simulink model "acc"  (R2020a)
settings: Solver=VariableStepAuto  StartTime=0.0  StopTime=inf  RelTol=1e-3
settings Model: Creator=shesh  LastModifiedBy=shesh

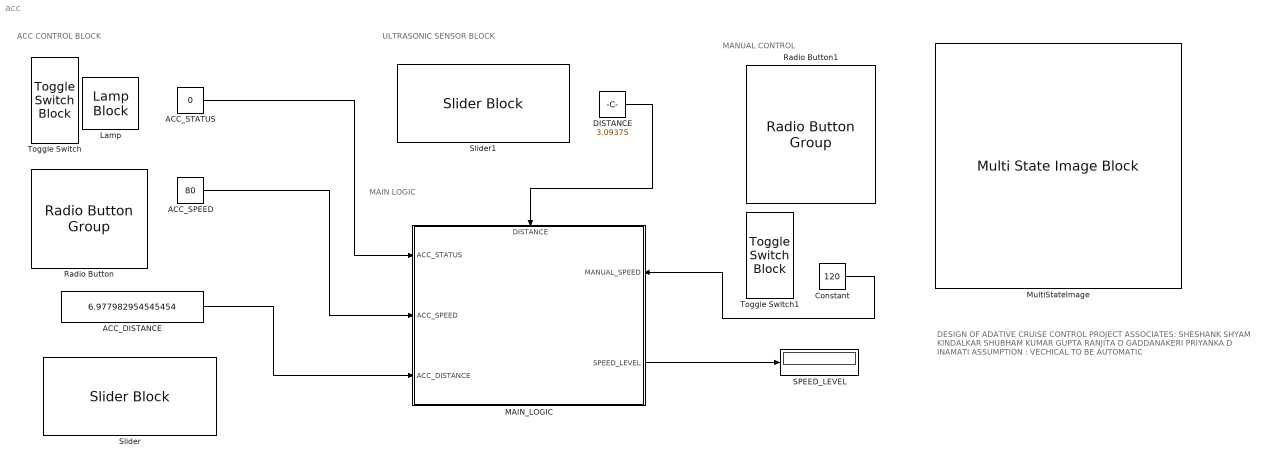
== system acc ==
  note: DESIGN OF ADATIVE CRUISE CONTROL
      |
      | PROJECT ASSOCIATES:
      | SHESHANK SHYAM KINDALKAR
      | SHUBHAM KUMAR GUPTA
      | RANJITA D GADDANAKERI
      | PRIYANKA D INAMATI
      |
      | ASSUMPTION : VECHICAL TO BE AUTOMATIC
  note: MANUAL CONTROL
  note: MAIN LOGIC
  note: ULTRASONIC SENSOR BLOCK
  note: ACC CONTROL BLOCK
  ACC_DISTANCE : Constant  Value=6.977982954545454  OutMin=[0]  OutMax=[10]
  ACC_SPEED : Constant  Value=80
  ACC_STATUS : Constant  Value=0
  Constant : Constant  Value=120
  DISTANCE : Constant  Value=3.09375
  Lamp : LampBlock
  MAIN_LOGIC : Stateflow chart  TreatAsAtomicUnit=on
      settings: PortSchema="{\"entries\":[{\"content\":{\"sides\":[{\"content\":{\"connectorIds\":[\"In3\",\"In4\",\"In5\"]},\"type\":\"ConnectorPlacement.EquallySpacedRectSide\",\"uuid\":\"9577933f-3cd5-4877-b3f1-1cabc5f66bc2\"},{\"content\":{\"connectorIds\":[\"In1\",\"Out1\"],\"side\":\"RIGHT\"},\"type\":\"ConnectorPlacement.EquallySpacedRectSide\",\"uuid\":\"2a6dc85d-fd72-47ef-ac66-14217eaecbf8\"},{\"content\":{\"connectorIds\":[\"In2\"],\"side\":\"TOP\"},\"type\":\"ConnectorPlacement.EquallySpacedRectSide\",\"uuid\":\"38d285f4-ccf6-4804-ae1f-6877806054a5\"}]},\"type\":\"ConnectorPlacement.EquallySpacedConnector\",\"uuid\":\"df4108ed-a8cc-4829-9830-7e09486e0f89\"}],\"packageUris\":[\"http://schema.mathworks.com/mf0/Connector/19700101\"],\"version\":\"1.0\"}"
  MultiStateImage : MultiStateImageBlock
  Radio Button : RadioButtonGroup  SelectedLabel=80 KMPH  ButtonGroupName=Group
      settings: Values={{'30 KMPH', '50 KMPH', '80 KMPH', '100 KMPH'}, [30 50 80 100]}
  Radio Button1 : RadioButtonGroup  SelectedLabel=120 KMPH  ButtonGroupName=Group
      settings: Values={{'40 KMPH', '80 KMPH', '120 KMPH', '160 KMPH', 'BREAK'}, [40 80 120 160 0]}
  SPEED_LEVEL : Display
  Slider : SliderBlock  ScaleMin=5  ScaleMax=10  TickInterval=1
  Slider1 : SliderBlock  ScaleMax=20
  Toggle Switch : ToggleSwitchBlock
      settings: Values={{'Off', 'On'}, [0 1]}
  Toggle Switch1 : ToggleSwitchBlock
      settings: Values={{'Off', 'On'}, [1 0]}
  wires:
  ACC_STATUS/1 -> MAIN_LOGIC/3(ACC_STATUS)
  ACC_SPEED/1 -> MAIN_LOGIC/4(ACC_SPEED)
  ACC_DISTANCE/1 -> MAIN_LOGIC/5(ACC_DISTANCE)
  DISTANCE/1 -> MAIN_LOGIC/2(DISTANCE)
  MAIN_LOGIC/1(SPEED_LEVEL) -> SPEED_LEVEL/1
  Constant/1 -> MAIN_LOGIC/1(MANUAL_SPEED)

== stateflow chart acc/MAIN_LOGIC ==
  state ADAPTIVE_CONTROL_ACTIVE
    entry:
    state ZERO_GEAR_STATE
      entry:
      SPEED_LEVEL = 0;
    state FRIST_GEAR_STATE
      entry:
      SPEED_LEVEL = 1;
    state SECOND_GEAR_STATE
      entry:
      SPEED_LEVEL = 2;
    state BREAKING_STATE
      entry:
      SPEED_LEVEL = 3;
    (default) -> ZERO_GEAR_STATE
    SECOND_GEAR_STATE -> FRIST_GEAR_STATE [order 5] : [ACC_SPEED == 80]
    ZERO_GEAR_STATE -> FRIST_GEAR_STATE [order 2] : [DISTANCE >= 0.20*ACC_DISTANCE]
    ZERO_GEAR_STATE -> ADAPTIVE_CONTROL_ACTIVE.BREAKING_STATE [order 1] : [DISTANCE >= 0.75*ACC_DISTANCE]
    FRIST_GEAR_STATE -> ZERO_GEAR_STATE [order 3] : [ACC_SPEED == 30 || ACC_SPEED == 50]
    ZERO_GEAR_STATE -> FRIST_GEAR_STATE [order 3] : [ACC_SPEED == 80]
    ADAPTIVE_CONTROL_ACTIVE.BREAKING_STATE -> FRIST_GEAR_STATE [order 4] : [ACC_SPEED == 80]
    FRIST_GEAR_STATE -> SECOND_GEAR_STATE [order 4] : [ACC_SPEED == 100]
    SECOND_GEAR_STATE -> ZERO_GEAR_STATE [order 4] : [ACC_SPEED == 30 || ACC_SPEED == 50]
    SECOND_GEAR_STATE -> ZERO_GEAR_STATE [order 2] : [DISTANCE >= 0.50*ACC_DISTANCE]
    ZERO_GEAR_STATE -> SECOND_GEAR_STATE [order 4] : [ACC_SPEED == 100]
    ADAPTIVE_CONTROL_ACTIVE.BREAKING_STATE -> ZERO_GEAR_STATE [order 1] : [DISTANCE >= 0.50*ACC_DISTANCE]
    ADAPTIVE_CONTROL_ACTIVE.BREAKING_STATE -> ZERO_GEAR_STATE [order 3] : [ACC_SPEED == 30 || ACC_SPEED == 50]
    FRIST_GEAR_STATE -> ZERO_GEAR_STATE [order 2] : [DISTANCE >= 0.50*ACC_DISTANCE]
    SECOND_GEAR_STATE -> FRIST_GEAR_STATE [order 3] : [DISTANCE >= 0.20*ACC_DISTANCE]
    FRIST_GEAR_STATE -> ADAPTIVE_CONTROL_ACTIVE.BREAKING_STATE [order 1] : [DISTANCE >= 0.75*ACC_DISTANCE]
    ADAPTIVE_CONTROL_ACTIVE.BREAKING_STATE -> FRIST_GEAR_STATE [order 2] : [DISTANCE >= 0.20*ACC_DISTANCE]
    SECOND_GEAR_STATE -> ADAPTIVE_CONTROL_ACTIVE.BREAKING_STATE [order 1] : [DISTANCE >= 0.75*ACC_DISTANCE]
    ADAPTIVE_CONTROL_ACTIVE.BREAKING_STATE -> SECOND_GEAR_STATE [order 5] : [ACC_SPEED == 100]
  state ADAPTIVE_CONTROL_INACTIVE
    entry:
    state SPEED_LEVEL_0
      entry:
      SPEED_LEVEL = 0;
    state SPEED_LEVEL_1
      entry:
      SPEED_LEVEL = 1;
    state SPEED_LEVEL_2
      entry:
      SPEED_LEVEL = 2;
    state BREAKING_STATE
      entry:
      SPEED_LEVEL = 3;
    SPEED_LEVEL_0 -> SPEED_LEVEL_1 [order 1] : [MANUAL_SPEED == 120]
    SPEED_LEVEL_1 -> SPEED_LEVEL_0 [order 3] : [(MANUAL_SPEED == 40) || (MANUAL_SPEED == 80)]
    (default) -> SPEED_LEVEL_0
    SPEED_LEVEL_0 -> ADAPTIVE_CONTROL_INACTIVE.BREAKING_STATE [order 3] : [MANUAL_SPEED == 160]
    SPEED_LEVEL_2 -> SPEED_LEVEL_1 [order 1] : [MANUAL_SPEED == 120]
    SPEED_LEVEL_2 -> SPEED_LEVEL_0 [order 3] : [(MANUAL_SPEED == 40) || (MANUAL_SPEED == 80)]
    SPEED_LEVEL_0 -> SPEED_LEVEL_2 [order 2] : [MANUAL_SPEED == 160]
    ADAPTIVE_CONTROL_INACTIVE.BREAKING_STATE -> SPEED_LEVEL_0 [order 3] : [(MANUAL_SPEED == 40) || (MANUAL_SPEED == 80)]
    SPEED_LEVEL_1 -> SPEED_LEVEL_2 [order 1] : [MANUAL_SPEED == 160]
    ADAPTIVE_CONTROL_INACTIVE.BREAKING_STATE -> SPEED_LEVEL_1 [order 1] : [MANUAL_SPEED == 120]
    SPEED_LEVEL_1 -> ADAPTIVE_CONTROL_INACTIVE.BREAKING_STATE [order 2] : [MANUAL_SPEED == 160]
    SPEED_LEVEL_2 -> ADAPTIVE_CONTROL_INACTIVE.BREAKING_STATE [order 2] : [MANUAL_SPEED == 160]
    ADAPTIVE_CONTROL_INACTIVE.BREAKING_STATE -> SPEED_LEVEL_2 [order 2] : [MANUAL_SPEED == 160]
  (default) -> ADAPTIVE_CONTROL_ACTIVE
  ADAPTIVE_CONTROL_ACTIVE -> ADAPTIVE_CONTROL_INACTIVE : [ACC_STATUS == 0]
  ADAPTIVE_CONTROL_INACTIVE -> ADAPTIVE_CONTROL_ACTIVE : [ACC_STATUS == 1]
  data: MANUAL_SPEED input; DISTANCE input; ACC_STATUS input; ACC_SPEED input; ACC_DISTANCE input; SPEED_LEVEL output
